simulink model "exp1"  (Simulink 7.6)
settings: Solver=ode45  StartTime=0.0  StopTime=15.0  RelTol=1e-3
undefined symbols (not defined in the file): kp
settings Model: Creator=pedro  LastModifiedBy=pedro
settings DataIOCC: LimitDataPoints=off

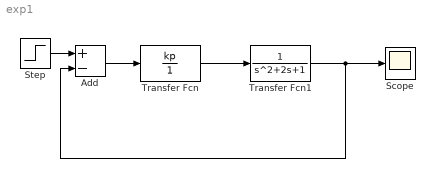
== system exp1 ==
  Add : Sum  Inputs=+-
  Scope : Scope
      settings: SampleInput=on  SampleTime=0.001
  Step : Step  Time=0  SampleTime=0
  Transfer Fcn : TransferFcn  Numerator=kp  Denominator=1
  Transfer Fcn1 : TransferFcn
  wires:
  Transfer Fcn1/1 -> Scope/1, Add/2
  Step/1 -> Add/1
  Transfer Fcn/1 -> Transfer Fcn1/1
  Add/1 -> Transfer Fcn/1
